simulink model "power_13NodeTestFeeder_4VSC_PV_DEG_symmtrc_loads_"  (R2024b)
settings: Solver=ode15s  StartTime=0.0  StopTime=5  FixedStep=1e-6  MaxStep=1e-4  RelTol=1e-6  AbsTol=1e-8  EnableMultiTasking=on
PreLoadFcn:
  | %power_13NodeTestFeeder_init;
values from neighbouring files (symbols this model uses):
  a = 1.3    [init_para_with_symmtrc_loads.m]
  Cdc = 278e-3    (= 0.278)    [init_para_with_symmtrc_loads.m]
  fg = 60    [a01_scan_VSC_13_feeder.m]    (also in init_para_with_symmtrc_loads.m)
  Gn = 1000    [init_para_with_symmtrc_loads.m]
  H = 8    [init_para_with_symmtrc_loads.m]
  Ipv_n = Isc_n*(Rp+Rs)/Rp    (= 8.21426513558)    [init_para_with_symmtrc_loads.m]
  Isc_n = 8.21    [init_para_with_symmtrc_loads.m]
  k = 1.3806503e-23    [init_para_with_symmtrc_loads.m]    (also in ypm_plot_compare_ana_meas.m = 2)
  Kdroop = Sn/(Rdroop*60)    (= 4166666.66667)    [init_para_with_symmtrc_loads.m]
  KI = 0.0032    [init_para_with_symmtrc_loads.m]
  Ki_C = Rc/tau_C    (= 0.768)    [init_para_with_symmtrc_loads.m]
  Ki_DC = omega_DC^2*Cdc    [init_para_with_symmtrc_loads.m]
  ki_dvpp = kp_dvpp/Ti_dvpp    [init_para_with_symmtrc_loads.m]
  Ki_P = 1/(Ki_pq*tau_P)    [init_para_with_symmtrc_loads.m]
  Ki_PLL = Kp_PLL/tau_PLL    [init_para_with_symmtrc_loads.m]
  Kp_C = Lc/tau_C    (= 0.020372)    [init_para_with_symmtrc_loads.m]
  Kp_DC = 2*xi_DC*omega_DC*Cdc    [init_para_with_symmtrc_loads.m]
  kp_dvpp = -(2*Kdcgain)^-1    [init_para_with_symmtrc_loads.m]
  Kp_P = tau_C/(Ki_pq*tau_P)    [init_para_with_symmtrc_loads.m]
  Kp_PLL = xi_PLL*2*omega_PLL/Vp    [init_para_with_symmtrc_loads.m]
  KV = -0.123    [init_para_with_symmtrc_loads.m]
  kv_Vp = [ 1.021 1.042 1.0174]    [init_para_with_symmtrc_loads.m]
  KVmp = Vmp_n/Voc_n    (= 0.799392097264)    [init_para_with_symmtrc_loads.m]
  Lc = 20.372e-6    (= 2.0372e-05)    [init_para_with_symmtrc_loads.m]
  Lg = Xg /(2*pi*fg)    [init_para_with_symmtrc_loads.m]
  Np = 345    [init_para_with_symmtrc_loads.m]
  Ns = 45    [init_para_with_symmtrc_loads.m]
  Ns_cell = 54    [init_para_with_symmtrc_loads.m]
  p_jump_time = 5    [init_para_with_symmtrc_loads.m]
  p_jump_value = 2*-1e6    (= -2000000)    [init_para_with_symmtrc_loads.m]
  phi_vec = phi_vec_deg/180*pi    [init_para_with_symmtrc_loads.m]
  ppv_nom = 4.9687e+05    (= 496870)    [init_para_with_symmtrc_loads.m]
  q = 1.6021764e-19    [init_para_with_symmtrc_loads.m]
  Rc = 0.768e-3    (= 0.000768)    [init_para_with_symmtrc_loads.m]
  Rg = (U_rms^2 / S_sc) / (sqrt(1 + XoverR^2))    [init_para_with_symmtrc_loads.m]
  Rp = 425.405    [init_para_with_symmtrc_loads.m]
  Rs = 0.221    [init_para_with_symmtrc_loads.m]
  S_base_all = 1    [init_para_with_symmtrc_loads.m]
  Sn = 15e6    (= 15000000)    [init_para_with_symmtrc_loads.m]
  tau_PLL = 2*xi_PLL/omega_PLL    [init_para_with_symmtrc_loads.m]
  Tn = 25    [init_para_with_symmtrc_loads.m]
  Ts = T_ctrl/n_ctrl    [a01_scan_VSC_13_feeder.m]    (also in init_para_with_symmtrc_loads.m = 5e-05)
  U_rms = 4160    [init_para_with_symmtrc_loads.m]
  Vdc = 1200    [init_para_with_symmtrc_loads.m]
  Voc_n = 32.9    [init_para_with_symmtrc_loads.m]
  Vp = sqrt(2)*480/sqrt(3)    [a01_scan_VSC_13_feeder.m]    (also in init_para_with_symmtrc_loads.m = Ug*sqrt(2)/sqrt(3))
undefined symbols (not defined in the file or in its folder): j, Newton, para_grid, para_PVgeno, Raphson
libraries: spsabctoAlphaBetaZeroLib x141, spsPower3phInstantaneousLib x70, spsSeriesRLCBranchLib x44, spsThreePhaseVIMeasurementLib x27, slpidlib x24, spsThreePhaseSeriesRLCLoadLib x15, spsControlledVoltageSourceLib x15, spsMeanLib x9, spsCurrentMeasurementLib x8, spsControlledCurrentSourceLib x8, cstblocks x8, spsGroundLib x5
(part 5 of 10)

== system power_13NodeTestFeeder_4VSC_PV_DEG_symmtrc_loads_/V I P Q Measurements EMT_with scopes_without_logsout/PQ_10 ==
  U : Inport
  I : Inport  Port=2
  Complex to Magnitude-Angle1 : ComplexToMagnitudeAngle
  Complex to Magnitude-Angle2 : ComplexToMagnitudeAngle
  Complex to Real-Imag : ComplexToRealImag
  Demux : Demux  Outputs=3
  Demux1 : Demux  Outputs=3
  Gain : Gain  Gain=1/S_base_all
  Gain1 : Gain  Gain=j
  Mux : Mux  Inputs=2
  "Power (3ph, Instantaneous)1" : spsPower3phInstantaneousLib/Power (3ph, Instantaneous)
  Real-Imag to Complex : RealImagToComplex
  Real-Imag to Complex1 : RealImagToComplex
  Sum : Sum  Inputs=|++
  Terminator{1,3,5..8} (6 alike) : Terminator
  Transfer Fcn{1..4} (4 alike) : TransferFcn  Denominator=[1e-3 1]
  abc to Alpha-Beta-Zero : spsabctoAlphaBetaZeroLib/abc to Alpha-Beta-Zero
  abc to Alpha-Beta-Zero1 : spsabctoAlphaBetaZeroLib/abc to Alpha-Beta-Zero
  PQ : Outport
  wires:
  I/1 -> abc to Alpha-Beta-Zero1/1, "Power (3ph, Instantaneous)1"/2
  Gain1/1 -> Sum/2
  Complex to Real-Imag/1 -> Mux/1
  Complex to Real-Imag/2 -> Mux/2
  Mux/1 -> PQ/1
  "Power (3ph, Instantaneous)1"/2 -> Transfer Fcn2/1
  "Power (3ph, Instantaneous)1"/1 -> Transfer Fcn1/1
  Sum/1 -> Gain/1
  Gain/1 -> Complex to Real-Imag/1
  U/1 -> abc to Alpha-Beta-Zero/1, "Power (3ph, Instantaneous)1"/1
  abc to Alpha-Beta-Zero/1 -> Demux/1
  Demux/1 -> Real-Imag to Complex/1
  Demux/2 -> Real-Imag to Complex/2
  Real-Imag to Complex/1 -> Complex to Magnitude-Angle2/1
  Complex to Magnitude-Angle2/1 -> Transfer Fcn3/1
  Complex to Magnitude-Angle2/2 -> Terminator3/1
  Complex to Magnitude-Angle1/1 -> Transfer Fcn4/1
  Real-Imag to Complex1/1 -> Complex to Magnitude-Angle1/1
  Demux1/2 -> Real-Imag to Complex1/2
  Demux1/1 -> Real-Imag to Complex1/1
  abc to Alpha-Beta-Zero1/1 -> Demux1/1
  Transfer Fcn1/1 -> Sum/1  "p"
  Transfer Fcn2/1 -> Gain1/1  "p"
  Transfer Fcn3/1 -> Terminator6/1  "u_betrag"
  Transfer Fcn4/1 -> Terminator5/1  "i_betrag"
  Demux1/3 -> Terminator7/1
  Demux/3 -> Terminator8/1
  Complex to Magnitude-Angle1/2 -> Terminator1/1

== system power_13NodeTestFeeder_4VSC_PV_DEG_symmtrc_loads_/V I P Q Measurements EMT_with scopes_without_logsout/PQ_11 ==
  U : Inport
  I : Inport  Port=2
  Complex to Magnitude-Angle1 : ComplexToMagnitudeAngle
  Complex to Magnitude-Angle2 : ComplexToMagnitudeAngle
  Complex to Real-Imag : ComplexToRealImag
  Demux : Demux  Outputs=3
  Demux1 : Demux  Outputs=3
  Gain : Gain  Gain=1/S_base_all
  Gain1 : Gain  Gain=j
  Mux : Mux  Inputs=2
  "Power (3ph, Instantaneous)1" : spsPower3phInstantaneousLib/Power (3ph, Instantaneous)
  Real-Imag to Complex : RealImagToComplex
  Real-Imag to Complex1 : RealImagToComplex
  Sum : Sum  Inputs=|++
  Terminator{1,3,5..8} (6 alike) : Terminator
  Transfer Fcn{1..4} (4 alike) : TransferFcn  Denominator=[1e-3 1]
  abc to Alpha-Beta-Zero : spsabctoAlphaBetaZeroLib/abc to Alpha-Beta-Zero
  abc to Alpha-Beta-Zero1 : spsabctoAlphaBetaZeroLib/abc to Alpha-Beta-Zero
  PQ : Outport
  wires:
  I/1 -> abc to Alpha-Beta-Zero1/1, "Power (3ph, Instantaneous)1"/2
  Gain1/1 -> Sum/2
  Complex to Real-Imag/1 -> Mux/1
  Complex to Real-Imag/2 -> Mux/2
  Mux/1 -> PQ/1
  "Power (3ph, Instantaneous)1"/2 -> Transfer Fcn2/1
  "Power (3ph, Instantaneous)1"/1 -> Transfer Fcn1/1
  Sum/1 -> Gain/1
  Gain/1 -> Complex to Real-Imag/1
  U/1 -> abc to Alpha-Beta-Zero/1, "Power (3ph, Instantaneous)1"/1
  abc to Alpha-Beta-Zero/1 -> Demux/1
  Demux/1 -> Real-Imag to Complex/1
  Demux/2 -> Real-Imag to Complex/2
  Real-Imag to Complex/1 -> Complex to Magnitude-Angle2/1
  Complex to Magnitude-Angle2/1 -> Transfer Fcn3/1
  Complex to Magnitude-Angle2/2 -> Terminator3/1
  Complex to Magnitude-Angle1/1 -> Transfer Fcn4/1
  Real-Imag to Complex1/1 -> Complex to Magnitude-Angle1/1
  Demux1/2 -> Real-Imag to Complex1/2
  Demux1/1 -> Real-Imag to Complex1/1
  abc to Alpha-Beta-Zero1/1 -> Demux1/1
  Transfer Fcn1/1 -> Sum/1  "p"
  Transfer Fcn2/1 -> Gain1/1  "p"
  Transfer Fcn3/1 -> Terminator6/1  "u_betrag"
  Transfer Fcn4/1 -> Terminator5/1  "i_betrag"
  Demux1/3 -> Terminator7/1
  Demux/3 -> Terminator8/1
  Complex to Magnitude-Angle1/2 -> Terminator1/1

== system power_13NodeTestFeeder_4VSC_PV_DEG_symmtrc_loads_/V I P Q Measurements EMT_with scopes_without_logsout/PQ_12 ==
  U : Inport
  I : Inport  Port=2
  Complex to Magnitude-Angle1 : ComplexToMagnitudeAngle
  Complex to Magnitude-Angle2 : ComplexToMagnitudeAngle
  Complex to Real-Imag : ComplexToRealImag
  Demux : Demux  Outputs=3
  Demux1 : Demux  Outputs=3
  Gain : Gain  Gain=1/S_base_all
  Gain1 : Gain  Gain=j
  Mux : Mux  Inputs=2
  "Power (3ph, Instantaneous)1" : spsPower3phInstantaneousLib/Power (3ph, Instantaneous)
  Real-Imag to Complex : RealImagToComplex
  Real-Imag to Complex1 : RealImagToComplex
  Sum : Sum  Inputs=|++
  Terminator{1,3,5..8} (6 alike) : Terminator
  Transfer Fcn{1..4} (4 alike) : TransferFcn  Denominator=[1e-3 1]
  abc to Alpha-Beta-Zero : spsabctoAlphaBetaZeroLib/abc to Alpha-Beta-Zero
  abc to Alpha-Beta-Zero1 : spsabctoAlphaBetaZeroLib/abc to Alpha-Beta-Zero
  PQ : Outport
  wires:
  I/1 -> abc to Alpha-Beta-Zero1/1, "Power (3ph, Instantaneous)1"/2
  Gain1/1 -> Sum/2
  Complex to Real-Imag/1 -> Mux/1
  Complex to Real-Imag/2 -> Mux/2
  Mux/1 -> PQ/1
  "Power (3ph, Instantaneous)1"/2 -> Transfer Fcn2/1
  "Power (3ph, Instantaneous)1"/1 -> Transfer Fcn1/1
  Sum/1 -> Gain/1
  Gain/1 -> Complex to Real-Imag/1
  U/1 -> abc to Alpha-Beta-Zero/1, "Power (3ph, Instantaneous)1"/1
  abc to Alpha-Beta-Zero/1 -> Demux/1
  Demux/1 -> Real-Imag to Complex/1
  Demux/2 -> Real-Imag to Complex/2
  Real-Imag to Complex/1 -> Complex to Magnitude-Angle2/1
  Complex to Magnitude-Angle2/1 -> Transfer Fcn3/1
  Complex to Magnitude-Angle2/2 -> Terminator3/1
  Complex to Magnitude-Angle1/1 -> Transfer Fcn4/1
  Real-Imag to Complex1/1 -> Complex to Magnitude-Angle1/1
  Demux1/2 -> Real-Imag to Complex1/2
  Demux1/1 -> Real-Imag to Complex1/1
  abc to Alpha-Beta-Zero1/1 -> Demux1/1
  Transfer Fcn1/1 -> Sum/1  "p"
  Transfer Fcn2/1 -> Gain1/1  "p"
  Transfer Fcn3/1 -> Terminator6/1  "u_betrag"
  Transfer Fcn4/1 -> Terminator5/1  "i_betrag"
  Demux1/3 -> Terminator7/1
  Demux/3 -> Terminator8/1
  Complex to Magnitude-Angle1/2 -> Terminator1/1

== system power_13NodeTestFeeder_4VSC_PV_DEG_symmtrc_loads_/V I P Q Measurements EMT_with scopes_without_logsout/PQ_13 ==
  U : Inport
  I : Inport  Port=2
  Complex to Magnitude-Angle1 : ComplexToMagnitudeAngle
  Complex to Magnitude-Angle2 : ComplexToMagnitudeAngle
  Complex to Real-Imag : ComplexToRealImag
  Demux : Demux  Outputs=3
  Demux1 : Demux  Outputs=3
  Gain : Gain  Gain=1/S_base_all
  Gain1 : Gain  Gain=j
  Mux : Mux  Inputs=2
  "Power (3ph, Instantaneous)1" : spsPower3phInstantaneousLib/Power (3ph, Instantaneous)
  Real-Imag to Complex : RealImagToComplex
  Real-Imag to Complex1 : RealImagToComplex
  Sum : Sum  Inputs=|++
  Terminator{1,3,5..8} (6 alike) : Terminator
  Transfer Fcn{1..4} (4 alike) : TransferFcn  Denominator=[1e-3 1]
  abc to Alpha-Beta-Zero : spsabctoAlphaBetaZeroLib/abc to Alpha-Beta-Zero
  abc to Alpha-Beta-Zero1 : spsabctoAlphaBetaZeroLib/abc to Alpha-Beta-Zero
  PQ : Outport
  wires:
  I/1 -> abc to Alpha-Beta-Zero1/1, "Power (3ph, Instantaneous)1"/2
  Gain1/1 -> Sum/2
  Complex to Real-Imag/1 -> Mux/1
  Complex to Real-Imag/2 -> Mux/2
  Mux/1 -> PQ/1
  "Power (3ph, Instantaneous)1"/2 -> Transfer Fcn2/1
  "Power (3ph, Instantaneous)1"/1 -> Transfer Fcn1/1
  Sum/1 -> Gain/1
  Gain/1 -> Complex to Real-Imag/1
  U/1 -> abc to Alpha-Beta-Zero/1, "Power (3ph, Instantaneous)1"/1
  abc to Alpha-Beta-Zero/1 -> Demux/1
  Demux/1 -> Real-Imag to Complex/1
  Demux/2 -> Real-Imag to Complex/2
  Real-Imag to Complex/1 -> Complex to Magnitude-Angle2/1
  Complex to Magnitude-Angle2/1 -> Transfer Fcn3/1
  Complex to Magnitude-Angle2/2 -> Terminator3/1
  Complex to Magnitude-Angle1/1 -> Transfer Fcn4/1
  Real-Imag to Complex1/1 -> Complex to Magnitude-Angle1/1
  Demux1/2 -> Real-Imag to Complex1/2
  Demux1/1 -> Real-Imag to Complex1/1
  abc to Alpha-Beta-Zero1/1 -> Demux1/1
  Transfer Fcn1/1 -> Sum/1  "p"
  Transfer Fcn2/1 -> Gain1/1  "p"
  Transfer Fcn3/1 -> Terminator6/1  "u_betrag"
  Transfer Fcn4/1 -> Terminator5/1  "i_betrag"
  Demux1/3 -> Terminator7/1
  Demux/3 -> Terminator8/1
  Complex to Magnitude-Angle1/2 -> Terminator1/1

== system power_13NodeTestFeeder_4VSC_PV_DEG_symmtrc_loads_/V I P Q Measurements EMT_with scopes_without_logsout/PQ_14 ==
  U : Inport
  I : Inport  Port=2
  Complex to Magnitude-Angle1 : ComplexToMagnitudeAngle
  Complex to Magnitude-Angle2 : ComplexToMagnitudeAngle
  Complex to Real-Imag : ComplexToRealImag
  Demux : Demux  Outputs=3
  Demux1 : Demux  Outputs=3
  Gain : Gain  Gain=1/S_base_all
  Gain1 : Gain  Gain=j
  Mux : Mux  Inputs=2
  "Power (3ph, Instantaneous)1" : spsPower3phInstantaneousLib/Power (3ph, Instantaneous)
  Real-Imag to Complex : RealImagToComplex
  Real-Imag to Complex1 : RealImagToComplex
  Sum : Sum  Inputs=|++
  Terminator{1,3,5..8} (6 alike) : Terminator
  Transfer Fcn{1..4} (4 alike) : TransferFcn  Denominator=[1e-3 1]
  abc to Alpha-Beta-Zero : spsabctoAlphaBetaZeroLib/abc to Alpha-Beta-Zero
  abc to Alpha-Beta-Zero1 : spsabctoAlphaBetaZeroLib/abc to Alpha-Beta-Zero
  PQ : Outport
  wires:
  I/1 -> abc to Alpha-Beta-Zero1/1, "Power (3ph, Instantaneous)1"/2
  Gain1/1 -> Sum/2
  Complex to Real-Imag/1 -> Mux/1
  Complex to Real-Imag/2 -> Mux/2
  Mux/1 -> PQ/1
  "Power (3ph, Instantaneous)1"/2 -> Transfer Fcn2/1
  "Power (3ph, Instantaneous)1"/1 -> Transfer Fcn1/1
  Sum/1 -> Gain/1
  Gain/1 -> Complex to Real-Imag/1
  U/1 -> abc to Alpha-Beta-Zero/1, "Power (3ph, Instantaneous)1"/1
  abc to Alpha-Beta-Zero/1 -> Demux/1
  Demux/1 -> Real-Imag to Complex/1
  Demux/2 -> Real-Imag to Complex/2
  Real-Imag to Complex/1 -> Complex to Magnitude-Angle2/1
  Complex to Magnitude-Angle2/1 -> Transfer Fcn3/1
  Complex to Magnitude-Angle2/2 -> Terminator3/1
  Complex to Magnitude-Angle1/1 -> Transfer Fcn4/1
  Real-Imag to Complex1/1 -> Complex to Magnitude-Angle1/1
  Demux1/2 -> Real-Imag to Complex1/2
  Demux1/1 -> Real-Imag to Complex1/1
  abc to Alpha-Beta-Zero1/1 -> Demux1/1
  Transfer Fcn1/1 -> Sum/1  "p"
  Transfer Fcn2/1 -> Gain1/1  "p"
  Transfer Fcn3/1 -> Terminator6/1  "u_betrag"
  Transfer Fcn4/1 -> Terminator5/1  "i_betrag"
  Demux1/3 -> Terminator7/1
  Demux/3 -> Terminator8/1
  Complex to Magnitude-Angle1/2 -> Terminator1/1

== system power_13NodeTestFeeder_4VSC_PV_DEG_symmtrc_loads_/V I P Q Measurements EMT_with scopes_without_logsout/PQ_15 ==
  U : Inport
  I : Inport  Port=2
  Complex to Magnitude-Angle1 : ComplexToMagnitudeAngle
  Complex to Magnitude-Angle2 : ComplexToMagnitudeAngle
  Complex to Real-Imag : ComplexToRealImag
  Demux : Demux  Outputs=3
  Demux1 : Demux  Outputs=3
  Gain : Gain  Gain=1/S_base_all
  Gain1 : Gain  Gain=j
  Mux : Mux  Inputs=2
  "Power (3ph, Instantaneous)1" : spsPower3phInstantaneousLib/Power (3ph, Instantaneous)
  Real-Imag to Complex : RealImagToComplex
  Real-Imag to Complex1 : RealImagToComplex
  Sum : Sum  Inputs=|++
  Terminator{1,3,5..8} (6 alike) : Terminator
  Transfer Fcn{1..4} (4 alike) : TransferFcn  Denominator=[1e-3 1]
  abc to Alpha-Beta-Zero : spsabctoAlphaBetaZeroLib/abc to Alpha-Beta-Zero
  abc to Alpha-Beta-Zero1 : spsabctoAlphaBetaZeroLib/abc to Alpha-Beta-Zero
  PQ : Outport
  wires:
  I/1 -> abc to Alpha-Beta-Zero1/1, "Power (3ph, Instantaneous)1"/2
  Gain1/1 -> Sum/2
  Complex to Real-Imag/1 -> Mux/1
  Complex to Real-Imag/2 -> Mux/2
  Mux/1 -> PQ/1
  "Power (3ph, Instantaneous)1"/2 -> Transfer Fcn2/1
  "Power (3ph, Instantaneous)1"/1 -> Transfer Fcn1/1
  Sum/1 -> Gain/1
  Gain/1 -> Complex to Real-Imag/1
  U/1 -> abc to Alpha-Beta-Zero/1, "Power (3ph, Instantaneous)1"/1
  abc to Alpha-Beta-Zero/1 -> Demux/1
  Demux/1 -> Real-Imag to Complex/1
  Demux/2 -> Real-Imag to Complex/2
  Real-Imag to Complex/1 -> Complex to Magnitude-Angle2/1
  Complex to Magnitude-Angle2/1 -> Transfer Fcn3/1
  Complex to Magnitude-Angle2/2 -> Terminator3/1
  Complex to Magnitude-Angle1/1 -> Transfer Fcn4/1
  Real-Imag to Complex1/1 -> Complex to Magnitude-Angle1/1
  Demux1/2 -> Real-Imag to Complex1/2
  Demux1/1 -> Real-Imag to Complex1/1
  abc to Alpha-Beta-Zero1/1 -> Demux1/1
  Transfer Fcn1/1 -> Sum/1  "p"
  Transfer Fcn2/1 -> Gain1/1  "p"
  Transfer Fcn3/1 -> Terminator6/1  "u_betrag"
  Transfer Fcn4/1 -> Terminator5/1  "i_betrag"
  Demux1/3 -> Terminator7/1
  Demux/3 -> Terminator8/1
  Complex to Magnitude-Angle1/2 -> Terminator1/1

== system power_13NodeTestFeeder_4VSC_PV_DEG_symmtrc_loads_/V I P Q Measurements EMT_with scopes_without_logsout/PQ_16 ==
  U : Inport
  I : Inport  Port=2
  Complex to Magnitude-Angle1 : ComplexToMagnitudeAngle
  Complex to Magnitude-Angle2 : ComplexToMagnitudeAngle
  Complex to Real-Imag : ComplexToRealImag
  Demux : Demux  Outputs=3
  Demux1 : Demux  Outputs=3
  Gain : Gain  Gain=1/S_base_all
  Gain1 : Gain  Gain=j
  Mux : Mux  Inputs=2
  "Power (3ph, Instantaneous)1" : spsPower3phInstantaneousLib/Power (3ph, Instantaneous)
  Real-Imag to Complex : RealImagToComplex
  Real-Imag to Complex1 : RealImagToComplex
  Sum : Sum  Inputs=|++
  Terminator{1,3,5..8} (6 alike) : Terminator
  Transfer Fcn{1..4} (4 alike) : TransferFcn  Denominator=[1e-3 1]
  abc to Alpha-Beta-Zero : spsabctoAlphaBetaZeroLib/abc to Alpha-Beta-Zero
  abc to Alpha-Beta-Zero1 : spsabctoAlphaBetaZeroLib/abc to Alpha-Beta-Zero
  PQ : Outport
  wires:
  I/1 -> abc to Alpha-Beta-Zero1/1, "Power (3ph, Instantaneous)1"/2
  Gain1/1 -> Sum/2
  Complex to Real-Imag/1 -> Mux/1
  Complex to Real-Imag/2 -> Mux/2
  Mux/1 -> PQ/1
  "Power (3ph, Instantaneous)1"/2 -> Transfer Fcn2/1
  "Power (3ph, Instantaneous)1"/1 -> Transfer Fcn1/1
  Sum/1 -> Gain/1
  Gain/1 -> Complex to Real-Imag/1
  U/1 -> abc to Alpha-Beta-Zero/1, "Power (3ph, Instantaneous)1"/1
  abc to Alpha-Beta-Zero/1 -> Demux/1
  Demux/1 -> Real-Imag to Complex/1
  Demux/2 -> Real-Imag to Complex/2
  Real-Imag to Complex/1 -> Complex to Magnitude-Angle2/1
  Complex to Magnitude-Angle2/1 -> Transfer Fcn3/1
  Complex to Magnitude-Angle2/2 -> Terminator3/1
  Complex to Magnitude-Angle1/1 -> Transfer Fcn4/1
  Real-Imag to Complex1/1 -> Complex to Magnitude-Angle1/1
  Demux1/2 -> Real-Imag to Complex1/2
  Demux1/1 -> Real-Imag to Complex1/1
  abc to Alpha-Beta-Zero1/1 -> Demux1/1
  Transfer Fcn1/1 -> Sum/1  "p"
  Transfer Fcn2/1 -> Gain1/1  "p"
  Transfer Fcn3/1 -> Terminator6/1  "u_betrag"
  Transfer Fcn4/1 -> Terminator5/1  "i_betrag"
  Demux1/3 -> Terminator7/1
  Demux/3 -> Terminator8/1
  Complex to Magnitude-Angle1/2 -> Terminator1/1

== system power_13NodeTestFeeder_4VSC_PV_DEG_symmtrc_loads_/V I P Q Measurements EMT_with scopes_without_logsout/PQ_17 ==
  U : Inport
  I : Inport  Port=2
  Complex to Magnitude-Angle1 : ComplexToMagnitudeAngle
  Complex to Magnitude-Angle2 : ComplexToMagnitudeAngle
  Complex to Real-Imag : ComplexToRealImag
  Demux : Demux  Outputs=3
  Demux1 : Demux  Outputs=3
  Gain : Gain  Gain=1/S_base_all
  Gain1 : Gain  Gain=j
  Mux : Mux  Inputs=2
  "Power (3ph, Instantaneous)1" : spsPower3phInstantaneousLib/Power (3ph, Instantaneous)
  Real-Imag to Complex : RealImagToComplex
  Real-Imag to Complex1 : RealImagToComplex
  Sum : Sum  Inputs=|++
  Terminator{1,3,5..8} (6 alike) : Terminator
  Transfer Fcn{1..4} (4 alike) : TransferFcn  Denominator=[1e-3 1]
  abc to Alpha-Beta-Zero : spsabctoAlphaBetaZeroLib/abc to Alpha-Beta-Zero
  abc to Alpha-Beta-Zero1 : spsabctoAlphaBetaZeroLib/abc to Alpha-Beta-Zero
  PQ : Outport
  wires:
  I/1 -> abc to Alpha-Beta-Zero1/1, "Power (3ph, Instantaneous)1"/2
  Gain1/1 -> Sum/2
  Complex to Real-Imag/1 -> Mux/1
  Complex to Real-Imag/2 -> Mux/2
  Mux/1 -> PQ/1
  "Power (3ph, Instantaneous)1"/2 -> Transfer Fcn2/1
  "Power (3ph, Instantaneous)1"/1 -> Transfer Fcn1/1
  Sum/1 -> Gain/1
  Gain/1 -> Complex to Real-Imag/1
  U/1 -> abc to Alpha-Beta-Zero/1, "Power (3ph, Instantaneous)1"/1
  abc to Alpha-Beta-Zero/1 -> Demux/1
  Demux/1 -> Real-Imag to Complex/1
  Demux/2 -> Real-Imag to Complex/2
  Real-Imag to Complex/1 -> Complex to Magnitude-Angle2/1
  Complex to Magnitude-Angle2/1 -> Transfer Fcn3/1
  Complex to Magnitude-Angle2/2 -> Terminator3/1
  Complex to Magnitude-Angle1/1 -> Transfer Fcn4/1
  Real-Imag to Complex1/1 -> Complex to Magnitude-Angle1/1
  Demux1/2 -> Real-Imag to Complex1/2
  Demux1/1 -> Real-Imag to Complex1/1
  abc to Alpha-Beta-Zero1/1 -> Demux1/1
  Transfer Fcn1/1 -> Sum/1  "p"
  Transfer Fcn2/1 -> Gain1/1  "p"
  Transfer Fcn3/1 -> Terminator6/1  "u_betrag"
  Transfer Fcn4/1 -> Terminator5/1  "i_betrag"
  Demux1/3 -> Terminator7/1
  Demux/3 -> Terminator8/1
  Complex to Magnitude-Angle1/2 -> Terminator1/1

== system power_13NodeTestFeeder_4VSC_PV_DEG_symmtrc_loads_/V I P Q Measurements EMT_with scopes_without_logsout/PQ_18 ==
  U : Inport
  I : Inport  Port=2
  Complex to Magnitude-Angle1 : ComplexToMagnitudeAngle
  Complex to Magnitude-Angle2 : ComplexToMagnitudeAngle
  Complex to Real-Imag : ComplexToRealImag
  Demux : Demux  Outputs=3
  Demux1 : Demux  Outputs=3
  Gain : Gain  Gain=1/S_base_all
  Gain1 : Gain  Gain=j
  Mux : Mux  Inputs=2
  "Power (3ph, Instantaneous)1" : spsPower3phInstantaneousLib/Power (3ph, Instantaneous)
  Real-Imag to Complex : RealImagToComplex
  Real-Imag to Complex1 : RealImagToComplex
  Sum : Sum  Inputs=|++
  Terminator{1,3,5..8} (6 alike) : Terminator
  Transfer Fcn{1..4} (4 alike) : TransferFcn  Denominator=[1e-3 1]
  abc to Alpha-Beta-Zero : spsabctoAlphaBetaZeroLib/abc to Alpha-Beta-Zero
  abc to Alpha-Beta-Zero1 : spsabctoAlphaBetaZeroLib/abc to Alpha-Beta-Zero
  PQ : Outport
  wires:
  I/1 -> abc to Alpha-Beta-Zero1/1, "Power (3ph, Instantaneous)1"/2
  Gain1/1 -> Sum/2
  Complex to Real-Imag/1 -> Mux/1
  Complex to Real-Imag/2 -> Mux/2
  Mux/1 -> PQ/1
  "Power (3ph, Instantaneous)1"/2 -> Transfer Fcn2/1
  "Power (3ph, Instantaneous)1"/1 -> Transfer Fcn1/1
  Sum/1 -> Gain/1
  Gain/1 -> Complex to Real-Imag/1
  U/1 -> abc to Alpha-Beta-Zero/1, "Power (3ph, Instantaneous)1"/1
  abc to Alpha-Beta-Zero/1 -> Demux/1
  Demux/1 -> Real-Imag to Complex/1
  Demux/2 -> Real-Imag to Complex/2
  Real-Imag to Complex/1 -> Complex to Magnitude-Angle2/1
  Complex to Magnitude-Angle2/1 -> Transfer Fcn3/1
  Complex to Magnitude-Angle2/2 -> Terminator3/1
  Complex to Magnitude-Angle1/1 -> Transfer Fcn4/1
  Real-Imag to Complex1/1 -> Complex to Magnitude-Angle1/1
  Demux1/2 -> Real-Imag to Complex1/2
  Demux1/1 -> Real-Imag to Complex1/1
  abc to Alpha-Beta-Zero1/1 -> Demux1/1
  Transfer Fcn1/1 -> Sum/1  "p"
  Transfer Fcn2/1 -> Gain1/1  "p"
  Transfer Fcn3/1 -> Terminator6/1  "u_betrag"
  Transfer Fcn4/1 -> Terminator5/1  "i_betrag"
  Demux1/3 -> Terminator7/1
  Demux/3 -> Terminator8/1
  Complex to Magnitude-Angle1/2 -> Terminator1/1

== system power_13NodeTestFeeder_4VSC_PV_DEG_symmtrc_loads_/V I P Q Measurements EMT_with scopes_without_logsout/PQ_19 ==
  U : Inport
  I : Inport  Port=2
  Complex to Magnitude-Angle1 : ComplexToMagnitudeAngle
  Complex to Magnitude-Angle2 : ComplexToMagnitudeAngle
  Complex to Real-Imag : ComplexToRealImag
  Demux : Demux  Outputs=3
  Demux1 : Demux  Outputs=3
  Gain : Gain  Gain=1/S_base_all
  Gain1 : Gain  Gain=j
  Mux : Mux  Inputs=2
  "Power (3ph, Instantaneous)1" : spsPower3phInstantaneousLib/Power (3ph, Instantaneous)
  Real-Imag to Complex : RealImagToComplex
  Real-Imag to Complex1 : RealImagToComplex
  Sum : Sum  Inputs=|++
  Terminator{1,3,5..8} (6 alike) : Terminator
  Transfer Fcn{1..4} (4 alike) : TransferFcn  Denominator=[1e-3 1]
  abc to Alpha-Beta-Zero : spsabctoAlphaBetaZeroLib/abc to Alpha-Beta-Zero
  abc to Alpha-Beta-Zero1 : spsabctoAlphaBetaZeroLib/abc to Alpha-Beta-Zero
  PQ : Outport
  wires:
  I/1 -> abc to Alpha-Beta-Zero1/1, "Power (3ph, Instantaneous)1"/2
  Gain1/1 -> Sum/2
  Complex to Real-Imag/1 -> Mux/1
  Complex to Real-Imag/2 -> Mux/2
  Mux/1 -> PQ/1
  "Power (3ph, Instantaneous)1"/2 -> Transfer Fcn2/1
  "Power (3ph, Instantaneous)1"/1 -> Transfer Fcn1/1
  Sum/1 -> Gain/1
  Gain/1 -> Complex to Real-Imag/1
  U/1 -> abc to Alpha-Beta-Zero/1, "Power (3ph, Instantaneous)1"/1
  abc to Alpha-Beta-Zero/1 -> Demux/1
  Demux/1 -> Real-Imag to Complex/1
  Demux/2 -> Real-Imag to Complex/2
  Real-Imag to Complex/1 -> Complex to Magnitude-Angle2/1
  Complex to Magnitude-Angle2/1 -> Transfer Fcn3/1
  Complex to Magnitude-Angle2/2 -> Terminator3/1
  Complex to Magnitude-Angle1/1 -> Transfer Fcn4/1
  Real-Imag to Complex1/1 -> Complex to Magnitude-Angle1/1
  Demux1/2 -> Real-Imag to Complex1/2
  Demux1/1 -> Real-Imag to Complex1/1
  abc to Alpha-Beta-Zero1/1 -> Demux1/1
  Transfer Fcn1/1 -> Sum/1  "p"
  Transfer Fcn2/1 -> Gain1/1  "p"
  Transfer Fcn3/1 -> Terminator6/1  "u_betrag"
  Transfer Fcn4/1 -> Terminator5/1  "i_betrag"
  Demux1/3 -> Terminator7/1
  Demux/3 -> Terminator8/1
  Complex to Magnitude-Angle1/2 -> Terminator1/1

== system power_13NodeTestFeeder_4VSC_PV_DEG_symmtrc_loads_/V I P Q Measurements EMT_with scopes_without_logsout/PQ_2 ==
  U : Inport
  I : Inport  Port=2
  Complex to Magnitude-Angle1 : ComplexToMagnitudeAngle
  Complex to Magnitude-Angle2 : ComplexToMagnitudeAngle
  Complex to Real-Imag : ComplexToRealImag
  Demux : Demux  Outputs=3
  Demux1 : Demux  Outputs=3
  Gain : Gain  Gain=1/S_base_all
  Gain1 : Gain  Gain=j
  Mux : Mux  Inputs=2
  "Power (3ph, Instantaneous)1" : spsPower3phInstantaneousLib/Power (3ph, Instantaneous)
  Real-Imag to Complex : RealImagToComplex
  Real-Imag to Complex1 : RealImagToComplex
  Sum : Sum  Inputs=|++
  Terminator{1,3,5..8} (6 alike) : Terminator
  Transfer Fcn{1..4} (4 alike) : TransferFcn  Denominator=[1e-3 1]
  abc to Alpha-Beta-Zero : spsabctoAlphaBetaZeroLib/abc to Alpha-Beta-Zero
  abc to Alpha-Beta-Zero1 : spsabctoAlphaBetaZeroLib/abc to Alpha-Beta-Zero
  PQ : Outport
  wires:
  I/1 -> abc to Alpha-Beta-Zero1/1, "Power (3ph, Instantaneous)1"/2
  Gain1/1 -> Sum/2
  Complex to Real-Imag/1 -> Mux/1
  Complex to Real-Imag/2 -> Mux/2
  Mux/1 -> PQ/1
  "Power (3ph, Instantaneous)1"/2 -> Transfer Fcn2/1
  "Power (3ph, Instantaneous)1"/1 -> Transfer Fcn1/1
  Sum/1 -> Gain/1
  Gain/1 -> Complex to Real-Imag/1
  U/1 -> abc to Alpha-Beta-Zero/1, "Power (3ph, Instantaneous)1"/1
  abc to Alpha-Beta-Zero/1 -> Demux/1
  Demux/1 -> Real-Imag to Complex/1
  Demux/2 -> Real-Imag to Complex/2
  Real-Imag to Complex/1 -> Complex to Magnitude-Angle2/1
  Complex to Magnitude-Angle2/1 -> Transfer Fcn3/1
  Complex to Magnitude-Angle2/2 -> Terminator3/1
  Complex to Magnitude-Angle1/1 -> Transfer Fcn4/1
  Real-Imag to Complex1/1 -> Complex to Magnitude-Angle1/1
  Demux1/2 -> Real-Imag to Complex1/2
  Demux1/1 -> Real-Imag to Complex1/1
  abc to Alpha-Beta-Zero1/1 -> Demux1/1
  Transfer Fcn1/1 -> Sum/1  "p"
  Transfer Fcn2/1 -> Gain1/1  "p"
  Transfer Fcn3/1 -> Terminator6/1  "u_betrag"
  Transfer Fcn4/1 -> Terminator5/1  "i_betrag"
  Demux1/3 -> Terminator7/1
  Demux/3 -> Terminator8/1
  Complex to Magnitude-Angle1/2 -> Terminator1/1

== system power_13NodeTestFeeder_4VSC_PV_DEG_symmtrc_loads_/V I P Q Measurements EMT_with scopes_without_logsout/PQ_3 ==
  U : Inport
  I : Inport  Port=2
  Complex to Magnitude-Angle1 : ComplexToMagnitudeAngle
  Complex to Magnitude-Angle2 : ComplexToMagnitudeAngle
  Complex to Real-Imag : ComplexToRealImag
  Demux : Demux  Outputs=3
  Demux1 : Demux  Outputs=3
  Gain : Gain  Gain=1/S_base_all
  Gain1 : Gain  Gain=j
  Mux : Mux  Inputs=2
  "Power (3ph, Instantaneous)1" : spsPower3phInstantaneousLib/Power (3ph, Instantaneous)
  Real-Imag to Complex : RealImagToComplex
  Real-Imag to Complex1 : RealImagToComplex
  Sum : Sum  Inputs=|++
  Terminator{1,3,5..8} (6 alike) : Terminator
  Transfer Fcn{1..4} (4 alike) : TransferFcn  Denominator=[1e-3 1]
  abc to Alpha-Beta-Zero : spsabctoAlphaBetaZeroLib/abc to Alpha-Beta-Zero
  abc to Alpha-Beta-Zero1 : spsabctoAlphaBetaZeroLib/abc to Alpha-Beta-Zero
  PQ : Outport
  wires:
  I/1 -> abc to Alpha-Beta-Zero1/1, "Power (3ph, Instantaneous)1"/2
  Gain1/1 -> Sum/2
  Complex to Real-Imag/1 -> Mux/1
  Complex to Real-Imag/2 -> Mux/2
  Mux/1 -> PQ/1
  "Power (3ph, Instantaneous)1"/2 -> Transfer Fcn2/1
  "Power (3ph, Instantaneous)1"/1 -> Transfer Fcn1/1
  Sum/1 -> Gain/1
  Gain/1 -> Complex to Real-Imag/1
  U/1 -> abc to Alpha-Beta-Zero/1, "Power (3ph, Instantaneous)1"/1
  abc to Alpha-Beta-Zero/1 -> Demux/1
  Demux/1 -> Real-Imag to Complex/1
  Demux/2 -> Real-Imag to Complex/2
  Real-Imag to Complex/1 -> Complex to Magnitude-Angle2/1
  Complex to Magnitude-Angle2/1 -> Transfer Fcn3/1
  Complex to Magnitude-Angle2/2 -> Terminator3/1
  Complex to Magnitude-Angle1/1 -> Transfer Fcn4/1
  Real-Imag to Complex1/1 -> Complex to Magnitude-Angle1/1
  Demux1/2 -> Real-Imag to Complex1/2
  Demux1/1 -> Real-Imag to Complex1/1
  abc to Alpha-Beta-Zero1/1 -> Demux1/1
  Transfer Fcn1/1 -> Sum/1  "p"
  Transfer Fcn2/1 -> Gain1/1  "p"
  Transfer Fcn3/1 -> Terminator6/1  "u_betrag"
  Transfer Fcn4/1 -> Terminator5/1  "i_betrag"
  Demux1/3 -> Terminator7/1
  Demux/3 -> Terminator8/1
  Complex to Magnitude-Angle1/2 -> Terminator1/1

== system power_13NodeTestFeeder_4VSC_PV_DEG_symmtrc_loads_/V I P Q Measurements EMT_with scopes_without_logsout/PQ_4 ==
  U : Inport
  I : Inport  Port=2
  Complex to Magnitude-Angle1 : ComplexToMagnitudeAngle
  Complex to Magnitude-Angle2 : ComplexToMagnitudeAngle
  Complex to Real-Imag : ComplexToRealImag
  Demux : Demux  Outputs=3
  Demux1 : Demux  Outputs=3
  Gain : Gain  Gain=1/S_base_all
  Gain1 : Gain  Gain=j
  Mux : Mux  Inputs=2
  "Power (3ph, Instantaneous)1" : spsPower3phInstantaneousLib/Power (3ph, Instantaneous)
  Real-Imag to Complex : RealImagToComplex
  Real-Imag to Complex1 : RealImagToComplex
  Sum : Sum  Inputs=|++
  Terminator{1,3,5..8} (6 alike) : Terminator
  Transfer Fcn{1..4} (4 alike) : TransferFcn  Denominator=[1e-3 1]
  abc to Alpha-Beta-Zero : spsabctoAlphaBetaZeroLib/abc to Alpha-Beta-Zero
  abc to Alpha-Beta-Zero1 : spsabctoAlphaBetaZeroLib/abc to Alpha-Beta-Zero
  PQ : Outport
  wires:
  I/1 -> abc to Alpha-Beta-Zero1/1, "Power (3ph, Instantaneous)1"/2
  Gain1/1 -> Sum/2
  Complex to Real-Imag/1 -> Mux/1
  Complex to Real-Imag/2 -> Mux/2
  Mux/1 -> PQ/1
  "Power (3ph, Instantaneous)1"/2 -> Transfer Fcn2/1
  "Power (3ph, Instantaneous)1"/1 -> Transfer Fcn1/1
  Sum/1 -> Gain/1
  Gain/1 -> Complex to Real-Imag/1
  U/1 -> abc to Alpha-Beta-Zero/1, "Power (3ph, Instantaneous)1"/1
  abc to Alpha-Beta-Zero/1 -> Demux/1
  Demux/1 -> Real-Imag to Complex/1
  Demux/2 -> Real-Imag to Complex/2
  Real-Imag to Complex/1 -> Complex to Magnitude-Angle2/1
  Complex to Magnitude-Angle2/1 -> Transfer Fcn3/1
  Complex to Magnitude-Angle2/2 -> Terminator3/1
  Complex to Magnitude-Angle1/1 -> Transfer Fcn4/1
  Real-Imag to Complex1/1 -> Complex to Magnitude-Angle1/1
  Demux1/2 -> Real-Imag to Complex1/2
  Demux1/1 -> Real-Imag to Complex1/1
  abc to Alpha-Beta-Zero1/1 -> Demux1/1
  Transfer Fcn1/1 -> Sum/1  "p"
  Transfer Fcn2/1 -> Gain1/1  "p"
  Transfer Fcn3/1 -> Terminator6/1  "u_betrag"
  Transfer Fcn4/1 -> Terminator5/1  "i_betrag"
  Demux1/3 -> Terminator7/1
  Demux/3 -> Terminator8/1
  Complex to Magnitude-Angle1/2 -> Terminator1/1

== system power_13NodeTestFeeder_4VSC_PV_DEG_symmtrc_loads_/V I P Q Measurements EMT_with scopes_without_logsout/PQ_5 ==
  U : Inport
  I : Inport  Port=2
  Complex to Magnitude-Angle1 : ComplexToMagnitudeAngle
  Complex to Magnitude-Angle2 : ComplexToMagnitudeAngle
  Complex to Real-Imag : ComplexToRealImag
  Demux : Demux  Outputs=3
  Demux1 : Demux  Outputs=3
  Gain : Gain  Gain=1/S_base_all
  Gain1 : Gain  Gain=j
  Mux : Mux  Inputs=2
  "Power (3ph, Instantaneous)1" : spsPower3phInstantaneousLib/Power (3ph, Instantaneous)
  Real-Imag to Complex : RealImagToComplex
  Real-Imag to Complex1 : RealImagToComplex
  Sum : Sum  Inputs=|++
  Terminator{1,3,5..8} (6 alike) : Terminator
  Transfer Fcn{1..4} (4 alike) : TransferFcn  Denominator=[1e-3 1]
  abc to Alpha-Beta-Zero : spsabctoAlphaBetaZeroLib/abc to Alpha-Beta-Zero
  abc to Alpha-Beta-Zero1 : spsabctoAlphaBetaZeroLib/abc to Alpha-Beta-Zero
  PQ : Outport
  wires:
  I/1 -> abc to Alpha-Beta-Zero1/1, "Power (3ph, Instantaneous)1"/2
  Gain1/1 -> Sum/2
  Complex to Real-Imag/1 -> Mux/1
  Complex to Real-Imag/2 -> Mux/2
  Mux/1 -> PQ/1
  "Power (3ph, Instantaneous)1"/2 -> Transfer Fcn2/1
  "Power (3ph, Instantaneous)1"/1 -> Transfer Fcn1/1
  Sum/1 -> Gain/1
  Gain/1 -> Complex to Real-Imag/1
  U/1 -> abc to Alpha-Beta-Zero/1, "Power (3ph, Instantaneous)1"/1
  abc to Alpha-Beta-Zero/1 -> Demux/1
  Demux/1 -> Real-Imag to Complex/1
  Demux/2 -> Real-Imag to Complex/2
  Real-Imag to Complex/1 -> Complex to Magnitude-Angle2/1
  Complex to Magnitude-Angle2/1 -> Transfer Fcn3/1
  Complex to Magnitude-Angle2/2 -> Terminator3/1
  Complex to Magnitude-Angle1/1 -> Transfer Fcn4/1
  Real-Imag to Complex1/1 -> Complex to Magnitude-Angle1/1
  Demux1/2 -> Real-Imag to Complex1/2
  Demux1/1 -> Real-Imag to Complex1/1
  abc to Alpha-Beta-Zero1/1 -> Demux1/1
  Transfer Fcn1/1 -> Sum/1  "p"
  Transfer Fcn2/1 -> Gain1/1  "p"
  Transfer Fcn3/1 -> Terminator6/1  "u_betrag"
  Transfer Fcn4/1 -> Terminator5/1  "i_betrag"
  Demux1/3 -> Terminator7/1
  Demux/3 -> Terminator8/1
  Complex to Magnitude-Angle1/2 -> Terminator1/1

== system power_13NodeTestFeeder_4VSC_PV_DEG_symmtrc_loads_/V I P Q Measurements EMT_with scopes_without_logsout/PQ_6 ==
  U : Inport
  I : Inport  Port=2
  Complex to Magnitude-Angle1 : ComplexToMagnitudeAngle
  Complex to Magnitude-Angle2 : ComplexToMagnitudeAngle
  Complex to Real-Imag : ComplexToRealImag
  Demux : Demux  Outputs=3
  Demux1 : Demux  Outputs=3
  Gain : Gain  Gain=1/S_base_all
  Gain1 : Gain  Gain=j
  Mux : Mux  Inputs=2
  "Power (3ph, Instantaneous)1" : spsPower3phInstantaneousLib/Power (3ph, Instantaneous)
  Real-Imag to Complex : RealImagToComplex
  Real-Imag to Complex1 : RealImagToComplex
  Sum : Sum  Inputs=|++
  Terminator{1,3,5..8} (6 alike) : Terminator
  Transfer Fcn{1..4} (4 alike) : TransferFcn  Denominator=[1e-3 1]
  abc to Alpha-Beta-Zero : spsabctoAlphaBetaZeroLib/abc to Alpha-Beta-Zero
  abc to Alpha-Beta-Zero1 : spsabctoAlphaBetaZeroLib/abc to Alpha-Beta-Zero
  PQ : Outport
  wires:
  I/1 -> abc to Alpha-Beta-Zero1/1, "Power (3ph, Instantaneous)1"/2
  Gain1/1 -> Sum/2
  Complex to Real-Imag/1 -> Mux/1
  Complex to Real-Imag/2 -> Mux/2
  Mux/1 -> PQ/1
  "Power (3ph, Instantaneous)1"/2 -> Transfer Fcn2/1
  "Power (3ph, Instantaneous)1"/1 -> Transfer Fcn1/1
  Sum/1 -> Gain/1
  Gain/1 -> Complex to Real-Imag/1
  U/1 -> abc to Alpha-Beta-Zero/1, "Power (3ph, Instantaneous)1"/1
  abc to Alpha-Beta-Zero/1 -> Demux/1
  Demux/1 -> Real-Imag to Complex/1
  Demux/2 -> Real-Imag to Complex/2
  Real-Imag to Complex/1 -> Complex to Magnitude-Angle2/1
  Complex to Magnitude-Angle2/1 -> Transfer Fcn3/1
  Complex to Magnitude-Angle2/2 -> Terminator3/1
  Complex to Magnitude-Angle1/1 -> Transfer Fcn4/1
  Real-Imag to Complex1/1 -> Complex to Magnitude-Angle1/1
  Demux1/2 -> Real-Imag to Complex1/2
  Demux1/1 -> Real-Imag to Complex1/1
  abc to Alpha-Beta-Zero1/1 -> Demux1/1
  Transfer Fcn1/1 -> Sum/1  "p"
  Transfer Fcn2/1 -> Gain1/1  "p"
  Transfer Fcn3/1 -> Terminator6/1  "u_betrag"
  Transfer Fcn4/1 -> Terminator5/1  "i_betrag"
  Demux1/3 -> Terminator7/1
  Demux/3 -> Terminator8/1
  Complex to Magnitude-Angle1/2 -> Terminator1/1

== system power_13NodeTestFeeder_4VSC_PV_DEG_symmtrc_loads_/V I P Q Measurements EMT_with scopes_without_logsout/PQ_7 ==
  U : Inport
  I : Inport  Port=2
  Complex to Magnitude-Angle1 : ComplexToMagnitudeAngle
  Complex to Magnitude-Angle2 : ComplexToMagnitudeAngle
  Complex to Real-Imag : ComplexToRealImag
  Demux : Demux  Outputs=3
  Demux1 : Demux  Outputs=3
  Gain : Gain  Gain=1/S_base_all
  Gain1 : Gain  Gain=j
  Mux : Mux  Inputs=2
  "Power (3ph, Instantaneous)1" : spsPower3phInstantaneousLib/Power (3ph, Instantaneous)
  Real-Imag to Complex : RealImagToComplex
  Real-Imag to Complex1 : RealImagToComplex
  Sum : Sum  Inputs=|++
  Terminator{1,3,5..8} (6 alike) : Terminator
  Transfer Fcn{1..4} (4 alike) : TransferFcn  Denominator=[1e-3 1]
  abc to Alpha-Beta-Zero : spsabctoAlphaBetaZeroLib/abc to Alpha-Beta-Zero
  abc to Alpha-Beta-Zero1 : spsabctoAlphaBetaZeroLib/abc to Alpha-Beta-Zero
  PQ : Outport
  wires:
  I/1 -> abc to Alpha-Beta-Zero1/1, "Power (3ph, Instantaneous)1"/2
  Gain1/1 -> Sum/2
  Complex to Real-Imag/1 -> Mux/1
  Complex to Real-Imag/2 -> Mux/2
  Mux/1 -> PQ/1
  "Power (3ph, Instantaneous)1"/2 -> Transfer Fcn2/1
  "Power (3ph, Instantaneous)1"/1 -> Transfer Fcn1/1
  Sum/1 -> Gain/1
  Gain/1 -> Complex to Real-Imag/1
  U/1 -> abc to Alpha-Beta-Zero/1, "Power (3ph, Instantaneous)1"/1
  abc to Alpha-Beta-Zero/1 -> Demux/1
  Demux/1 -> Real-Imag to Complex/1
  Demux/2 -> Real-Imag to Complex/2
  Real-Imag to Complex/1 -> Complex to Magnitude-Angle2/1
  Complex to Magnitude-Angle2/1 -> Transfer Fcn3/1
  Complex to Magnitude-Angle2/2 -> Terminator3/1
  Complex to Magnitude-Angle1/1 -> Transfer Fcn4/1
  Real-Imag to Complex1/1 -> Complex to Magnitude-Angle1/1
  Demux1/2 -> Real-Imag to Complex1/2
  Demux1/1 -> Real-Imag to Complex1/1
  abc to Alpha-Beta-Zero1/1 -> Demux1/1
  Transfer Fcn1/1 -> Sum/1  "p"
  Transfer Fcn2/1 -> Gain1/1  "p"
  Transfer Fcn3/1 -> Terminator6/1  "u_betrag"
  Transfer Fcn4/1 -> Terminator5/1  "i_betrag"
  Demux1/3 -> Terminator7/1
  Demux/3 -> Terminator8/1
  Complex to Magnitude-Angle1/2 -> Terminator1/1

== system power_13NodeTestFeeder_4VSC_PV_DEG_symmtrc_loads_/V I P Q Measurements EMT_with scopes_without_logsout/PQ_8 ==
  U : Inport
  I : Inport  Port=2
  Complex to Magnitude-Angle1 : ComplexToMagnitudeAngle
  Complex to Magnitude-Angle2 : ComplexToMagnitudeAngle
  Complex to Real-Imag : ComplexToRealImag
  Demux : Demux  Outputs=3
  Demux1 : Demux  Outputs=3
  Gain : Gain  Gain=1/S_base_all
  Gain1 : Gain  Gain=j
  Mux : Mux  Inputs=2
  "Power (3ph, Instantaneous)1" : spsPower3phInstantaneousLib/Power (3ph, Instantaneous)
  Real-Imag to Complex : RealImagToComplex
  Real-Imag to Complex1 : RealImagToComplex
  Sum : Sum  Inputs=|++
  Terminator{1,3,5..8} (6 alike) : Terminator
  Transfer Fcn{1..4} (4 alike) : TransferFcn  Denominator=[1e-3 1]
  abc to Alpha-Beta-Zero : spsabctoAlphaBetaZeroLib/abc to Alpha-Beta-Zero
  abc to Alpha-Beta-Zero1 : spsabctoAlphaBetaZeroLib/abc to Alpha-Beta-Zero
  PQ : Outport
  wires:
  I/1 -> abc to Alpha-Beta-Zero1/1, "Power (3ph, Instantaneous)1"/2
  Gain1/1 -> Sum/2
  Complex to Real-Imag/1 -> Mux/1
  Complex to Real-Imag/2 -> Mux/2
  Mux/1 -> PQ/1
  "Power (3ph, Instantaneous)1"/2 -> Transfer Fcn2/1
  "Power (3ph, Instantaneous)1"/1 -> Transfer Fcn1/1
  Sum/1 -> Gain/1
  Gain/1 -> Complex to Real-Imag/1
  U/1 -> abc to Alpha-Beta-Zero/1, "Power (3ph, Instantaneous)1"/1
  abc to Alpha-Beta-Zero/1 -> Demux/1
  Demux/1 -> Real-Imag to Complex/1
  Demux/2 -> Real-Imag to Complex/2
  Real-Imag to Complex/1 -> Complex to Magnitude-Angle2/1
  Complex to Magnitude-Angle2/1 -> Transfer Fcn3/1
  Complex to Magnitude-Angle2/2 -> Terminator3/1
  Complex to Magnitude-Angle1/1 -> Transfer Fcn4/1
  Real-Imag to Complex1/1 -> Complex to Magnitude-Angle1/1
  Demux1/2 -> Real-Imag to Complex1/2
  Demux1/1 -> Real-Imag to Complex1/1
  abc to Alpha-Beta-Zero1/1 -> Demux1/1
  Transfer Fcn1/1 -> Sum/1  "p"
  Transfer Fcn2/1 -> Gain1/1  "p"
  Transfer Fcn3/1 -> Terminator6/1  "u_betrag"
  Transfer Fcn4/1 -> Terminator5/1  "i_betrag"
  Demux1/3 -> Terminator7/1
  Demux/3 -> Terminator8/1
  Complex to Magnitude-Angle1/2 -> Terminator1/1

== system power_13NodeTestFeeder_4VSC_PV_DEG_symmtrc_loads_/V I P Q Measurements EMT_with scopes_without_logsout/PQ_9 ==
  U : Inport
  I : Inport  Port=2
  Complex to Magnitude-Angle1 : ComplexToMagnitudeAngle
  Complex to Magnitude-Angle2 : ComplexToMagnitudeAngle
  Complex to Real-Imag : ComplexToRealImag
  Demux : Demux  Outputs=3
  Demux1 : Demux  Outputs=3
  Gain : Gain  Gain=1/S_base_all
  Gain1 : Gain  Gain=j
  Mux : Mux  Inputs=2
  "Power (3ph, Instantaneous)1" : spsPower3phInstantaneousLib/Power (3ph, Instantaneous)
  Real-Imag to Complex : RealImagToComplex
  Real-Imag to Complex1 : RealImagToComplex
  Sum : Sum  Inputs=|++
  Terminator{1,3,5..8} (6 alike) : Terminator
  Transfer Fcn{1..4} (4 alike) : TransferFcn  Denominator=[1e-3 1]
  abc to Alpha-Beta-Zero : spsabctoAlphaBetaZeroLib/abc to Alpha-Beta-Zero
  abc to Alpha-Beta-Zero1 : spsabctoAlphaBetaZeroLib/abc to Alpha-Beta-Zero
  PQ : Outport
  wires:
  I/1 -> abc to Alpha-Beta-Zero1/1, "Power (3ph, Instantaneous)1"/2
  Gain1/1 -> Sum/2
  Complex to Real-Imag/1 -> Mux/1
  Complex to Real-Imag/2 -> Mux/2
  Mux/1 -> PQ/1
  "Power (3ph, Instantaneous)1"/2 -> Transfer Fcn2/1
  "Power (3ph, Instantaneous)1"/1 -> Transfer Fcn1/1
  Sum/1 -> Gain/1
  Gain/1 -> Complex to Real-Imag/1
  U/1 -> abc to Alpha-Beta-Zero/1, "Power (3ph, Instantaneous)1"/1
  abc to Alpha-Beta-Zero/1 -> Demux/1
  Demux/1 -> Real-Imag to Complex/1
  Demux/2 -> Real-Imag to Complex/2
  Real-Imag to Complex/1 -> Complex to Magnitude-Angle2/1
  Complex to Magnitude-Angle2/1 -> Transfer Fcn3/1
  Complex to Magnitude-Angle2/2 -> Terminator3/1
  Complex to Magnitude-Angle1/1 -> Transfer Fcn4/1
  Real-Imag to Complex1/1 -> Complex to Magnitude-Angle1/1
  Demux1/2 -> Real-Imag to Complex1/2
  Demux1/1 -> Real-Imag to Complex1/1
  abc to Alpha-Beta-Zero1/1 -> Demux1/1
  Transfer Fcn1/1 -> Sum/1  "p"
  Transfer Fcn2/1 -> Gain1/1  "p"
  Transfer Fcn3/1 -> Terminator6/1  "u_betrag"
  Transfer Fcn4/1 -> Terminator5/1  "i_betrag"
  Demux1/3 -> Terminator7/1
  Demux/3 -> Terminator8/1
  Complex to Magnitude-Angle1/2 -> Terminator1/1

== system power_13NodeTestFeeder_4VSC_PV_DEG_symmtrc_loads_/V I P Q Measurements EMT_with scopes_without_logsout/Subsystem3 ==
  In1 : Inport
  Gain : Gain  Gain=1/3
  Mean value : spsMeanLib/Mean  Freq=fg  Vinit=Vrms0  Ts=Ts
  Product : Product  InputSameDT=on  SaturateOnIntegerOverflow=on  OutDataTypeStr=Inherit: Same as first input
  Saturation to avoid negative sqrt : Saturate  UpperLimit=Inf  LowerLimit=0
  Sqrt : Sqrt  AlgorithmType=Newton-Raphson
  Sum of Elements : Sum  Inputs=+
  Out1 : Outport
  wires:
  Sqrt/1 -> Sum of Elements/1
  Mean value/1 -> Saturation to avoid negative sqrt/1
  Saturation to avoid negative sqrt/1 -> Sqrt/1
  Product/1 -> Mean value/1
  In1/1 -> Product/2, Product/1
  Sum of Elements/1 -> Gain/1
  Gain/1 -> Out1/1

== system power_13NodeTestFeeder_4VSC_PV_DEG_symmtrc_loads_/V I P Q Measurements EMT_without scopes_with_logsout/PQ_1 ==
  U : Inport
  I : Inport  Port=2
  Complex to Magnitude-Angle1 : ComplexToMagnitudeAngle
  Complex to Magnitude-Angle2 : ComplexToMagnitudeAngle
  Complex to Real-Imag : ComplexToRealImag
  Demux : Demux  Outputs=3
  Demux1 : Demux  Outputs=3
  Gain : Gain  Gain=1/S_base_all
  Gain1 : Gain  Gain=j
  Mux : Mux  Inputs=2
  "Power (3ph, Instantaneous)1" : spsPower3phInstantaneousLib/Power (3ph, Instantaneous)
  Real-Imag to Complex : RealImagToComplex
  Real-Imag to Complex1 : RealImagToComplex
  Sum : Sum  Inputs=|++
  Terminator{1,3,5..8} (6 alike) : Terminator
  Transfer Fcn{1..4} (4 alike) : TransferFcn  Denominator=[1e-3 1]
  abc to Alpha-Beta-Zero : spsabctoAlphaBetaZeroLib/abc to Alpha-Beta-Zero
  abc to Alpha-Beta-Zero1 : spsabctoAlphaBetaZeroLib/abc to Alpha-Beta-Zero
  PQ : Outport
  wires:
  I/1 -> abc to Alpha-Beta-Zero1/1, "Power (3ph, Instantaneous)1"/2
  Gain1/1 -> Sum/2
  Complex to Real-Imag/1 -> Mux/1
  Complex to Real-Imag/2 -> Mux/2
  Mux/1 -> PQ/1
  "Power (3ph, Instantaneous)1"/2 -> Transfer Fcn2/1
  "Power (3ph, Instantaneous)1"/1 -> Transfer Fcn1/1
  Sum/1 -> Gain/1
  Gain/1 -> Complex to Real-Imag/1
  U/1 -> abc to Alpha-Beta-Zero/1, "Power (3ph, Instantaneous)1"/1
  abc to Alpha-Beta-Zero/1 -> Demux/1
  Demux/1 -> Real-Imag to Complex/1
  Demux/2 -> Real-Imag to Complex/2
  Real-Imag to Complex/1 -> Complex to Magnitude-Angle2/1
  Complex to Magnitude-Angle2/1 -> Transfer Fcn3/1
  Complex to Magnitude-Angle2/2 -> Terminator3/1
  Complex to Magnitude-Angle1/1 -> Transfer Fcn4/1
  Real-Imag to Complex1/1 -> Complex to Magnitude-Angle1/1
  Demux1/2 -> Real-Imag to Complex1/2
  Demux1/1 -> Real-Imag to Complex1/1
  abc to Alpha-Beta-Zero1/1 -> Demux1/1
  Transfer Fcn1/1 -> Sum/1  "p"
  Transfer Fcn2/1 -> Gain1/1  "p"
  Transfer Fcn3/1 -> Terminator6/1  "u_betrag"
  Transfer Fcn4/1 -> Terminator5/1  "i_betrag"
  Demux1/3 -> Terminator7/1
  Demux/3 -> Terminator8/1
  Complex to Magnitude-Angle1/2 -> Terminator1/1

== system power_13NodeTestFeeder_4VSC_PV_DEG_symmtrc_loads_/V I P Q Measurements EMT_without scopes_with_logsout/PQ_10 ==
  U : Inport
  I : Inport  Port=2
  Complex to Magnitude-Angle1 : ComplexToMagnitudeAngle
  Complex to Magnitude-Angle2 : ComplexToMagnitudeAngle
  Complex to Real-Imag : ComplexToRealImag
  Demux : Demux  Outputs=3
  Demux1 : Demux  Outputs=3
  Gain : Gain  Gain=1/S_base_all
  Gain1 : Gain  Gain=j
  Mux : Mux  Inputs=2
  "Power (3ph, Instantaneous)1" : spsPower3phInstantaneousLib/Power (3ph, Instantaneous)
  Real-Imag to Complex : RealImagToComplex
  Real-Imag to Complex1 : RealImagToComplex
  Sum : Sum  Inputs=|++
  Terminator{1,3,5..8} (6 alike) : Terminator
  Transfer Fcn{1..4} (4 alike) : TransferFcn  Denominator=[1e-3 1]
  abc to Alpha-Beta-Zero : spsabctoAlphaBetaZeroLib/abc to Alpha-Beta-Zero
  abc to Alpha-Beta-Zero1 : spsabctoAlphaBetaZeroLib/abc to Alpha-Beta-Zero
  PQ : Outport
  wires:
  I/1 -> abc to Alpha-Beta-Zero1/1, "Power (3ph, Instantaneous)1"/2
  Gain1/1 -> Sum/2
  Complex to Real-Imag/1 -> Mux/1
  Complex to Real-Imag/2 -> Mux/2
  Mux/1 -> PQ/1
  "Power (3ph, Instantaneous)1"/2 -> Transfer Fcn2/1
  "Power (3ph, Instantaneous)1"/1 -> Transfer Fcn1/1
  Sum/1 -> Gain/1
  Gain/1 -> Complex to Real-Imag/1
  U/1 -> abc to Alpha-Beta-Zero/1, "Power (3ph, Instantaneous)1"/1
  abc to Alpha-Beta-Zero/1 -> Demux/1
  Demux/1 -> Real-Imag to Complex/1
  Demux/2 -> Real-Imag to Complex/2
  Real-Imag to Complex/1 -> Complex to Magnitude-Angle2/1
  Complex to Magnitude-Angle2/1 -> Transfer Fcn3/1
  Complex to Magnitude-Angle2/2 -> Terminator3/1
  Complex to Magnitude-Angle1/1 -> Transfer Fcn4/1
  Real-Imag to Complex1/1 -> Complex to Magnitude-Angle1/1
  Demux1/2 -> Real-Imag to Complex1/2
  Demux1/1 -> Real-Imag to Complex1/1
  abc to Alpha-Beta-Zero1/1 -> Demux1/1
  Transfer Fcn1/1 -> Sum/1  "p"
  Transfer Fcn2/1 -> Gain1/1  "p"
  Transfer Fcn3/1 -> Terminator6/1  "u_betrag"
  Transfer Fcn4/1 -> Terminator5/1  "i_betrag"
  Demux1/3 -> Terminator7/1
  Demux/3 -> Terminator8/1
  Complex to Magnitude-Angle1/2 -> Terminator1/1

== system power_13NodeTestFeeder_4VSC_PV_DEG_symmtrc_loads_/V I P Q Measurements EMT_without scopes_with_logsout/PQ_11 ==
  U : Inport
  I : Inport  Port=2
  Complex to Magnitude-Angle1 : ComplexToMagnitudeAngle
  Complex to Magnitude-Angle2 : ComplexToMagnitudeAngle
  Complex to Real-Imag : ComplexToRealImag
  Demux : Demux  Outputs=3
  Demux1 : Demux  Outputs=3
  Gain : Gain  Gain=1/S_base_all
  Gain1 : Gain  Gain=j
  Mux : Mux  Inputs=2
  "Power (3ph, Instantaneous)1" : spsPower3phInstantaneousLib/Power (3ph, Instantaneous)
  Real-Imag to Complex : RealImagToComplex
  Real-Imag to Complex1 : RealImagToComplex
  Sum : Sum  Inputs=|++
  Terminator{1,3,5..8} (6 alike) : Terminator
  Transfer Fcn{1..4} (4 alike) : TransferFcn  Denominator=[1e-3 1]
  abc to Alpha-Beta-Zero : spsabctoAlphaBetaZeroLib/abc to Alpha-Beta-Zero
  abc to Alpha-Beta-Zero1 : spsabctoAlphaBetaZeroLib/abc to Alpha-Beta-Zero
  PQ : Outport
  wires:
  I/1 -> abc to Alpha-Beta-Zero1/1, "Power (3ph, Instantaneous)1"/2
  Gain1/1 -> Sum/2
  Complex to Real-Imag/1 -> Mux/1
  Complex to Real-Imag/2 -> Mux/2
  Mux/1 -> PQ/1
  "Power (3ph, Instantaneous)1"/2 -> Transfer Fcn2/1
  "Power (3ph, Instantaneous)1"/1 -> Transfer Fcn1/1
  Sum/1 -> Gain/1
  Gain/1 -> Complex to Real-Imag/1
  U/1 -> abc to Alpha-Beta-Zero/1, "Power (3ph, Instantaneous)1"/1
  abc to Alpha-Beta-Zero/1 -> Demux/1
  Demux/1 -> Real-Imag to Complex/1
  Demux/2 -> Real-Imag to Complex/2
  Real-Imag to Complex/1 -> Complex to Magnitude-Angle2/1
  Complex to Magnitude-Angle2/1 -> Transfer Fcn3/1
  Complex to Magnitude-Angle2/2 -> Terminator3/1
  Complex to Magnitude-Angle1/1 -> Transfer Fcn4/1
  Real-Imag to Complex1/1 -> Complex to Magnitude-Angle1/1
  Demux1/2 -> Real-Imag to Complex1/2
  Demux1/1 -> Real-Imag to Complex1/1
  abc to Alpha-Beta-Zero1/1 -> Demux1/1
  Transfer Fcn1/1 -> Sum/1  "p"
  Transfer Fcn2/1 -> Gain1/1  "p"
  Transfer Fcn3/1 -> Terminator6/1  "u_betrag"
  Transfer Fcn4/1 -> Terminator5/1  "i_betrag"
  Demux1/3 -> Terminator7/1
  Demux/3 -> Terminator8/1
  Complex to Magnitude-Angle1/2 -> Terminator1/1
